simulink model "VDB_Unreal_ClosedLoop"  (R2026b)
settings: Solver=ode4  StopTime=35  FixedStep=0.02
undefined symbols (not defined in the file or in its folder): sih
libraries: sim3dlib x1, sim3dautolib x1, sim3dcameralib x1, autolibshared x1
settings Model: Creator=Hp  LastModifiedBy=Hp

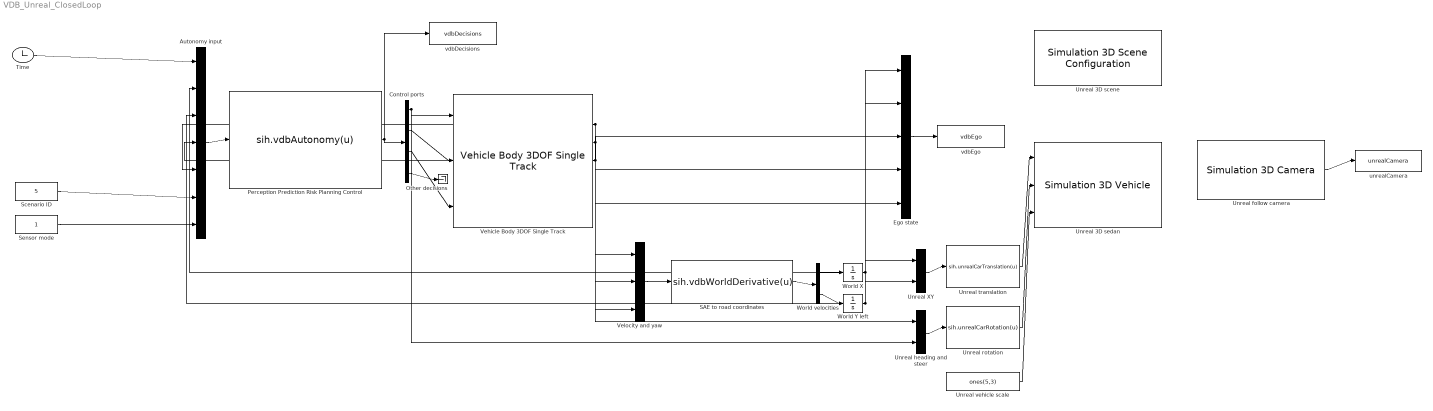
== system VDB_Unreal_ClosedLoop ==
  Autonomy input : Mux  Inputs=7
  Control ports : Demux  Outputs=[1 1 1 27]
  Ego state : Mux  Inputs=5
  Other decisions : Terminator
  Perception Prediction Risk Planning Control : MATLABFcn  MATLABFcn=sih.vdbAutonomy(u)  OutputDimensions=30  SampleTime=0.1
  SAE to road coordinates : MATLABFcn  MATLABFcn=sih.vdbWorldDerivative(u)  OutputDimensions=2  SampleTime=0.02
  Scenario ID : Constant  Value=5
  Sensor mode : Constant
  Time : Clock
  Unreal 3D scene : sim3dlib/Simulation 3D Scene Configuration  Priority=0  EnableWindow=on  ViewerType=Default Viewer  ProjectFormat=Default Scenes  SceneDesc=Open surface  ProjectName=C:\Program Files\MATLAB\R2026b\toolbox\shared\sim3d_projects\automotive_project_windows\UE\WindowsNoEditor\VehicleSimulation.exe  ScenePath=/Game/Maps/HwStrght  EnableOpenDRIVE=off  vehTagList={'Custom';'Scene Origin'}  vehTag=Custom  AttachedCameraRelativeTranslation=[0 0 0]  FreeCameraDefaultInitialTranslation=[-6, 0, 2]  AttachedCameraRelativeRotation=[0, -15, 0]  FreeCameraDefaultInitialRotation=[0, -15, 0]  ViewpointName=Custom  FreeCameraInitialTranslation=[0 0 0]  FreeCameraInitialRotation=[0 0 0]  OpVisEn=off  Ts=.02  EnableRemoteAccess=off  SimulationMode=CoSimulation  SimulateUsing=Interpreted execution  EnableAnimationRecording=off  OverrideDefaultRecording=off  AnimationRecordingFileName=sim3dAnimation.mat  AnimationRecordingInterval=[0 inf]  EnableWeather=off  SunAzimuth=90  SunAltitude=40.0  EnableGeospatialSun=off  Latitude=0  Longitude=0  Date=2023-01-01  Time=10:30:00  GeoTimeZone=-5.0  SunDaylightSaving=off  wind=1  clouds=10  EnableVolumetricClouds=off  CloudCoverage=0  CloudAltitude=6  fog=0  rain=0  RaindropsEffect=off  SnowDensity=0  EnableGeospatial=off  TilesetSource=Earth terrain  UseTrueOrigin=off  OriginHeight=200  OriginLatitude=40.744652  OriginLongitude=-73.988864  MapStyle=Aerial  AdditionalAssetIDs=[]  UseAdvancedSunSky=off  SolarTime=11  TimeZone=-5  Day=21  Month=9  Year=2022  UseDaylightSavingTime=on  DSTStartDay=10  DSTStartMonth=3  DSTEndDay=3  DSTEndMonth=11  DSTSwitchHour=2  sensorTag=MainCamera1  sensorId=1  sensorName=MainCamera1  mountLoc=Origin  offsetFlag=off  tmountOffset=[0, 0, 0]  rmountOffset=[0, 0, 0]  HorizontalResolution=1280  VerticalResolution=720  HorizontalFOV=60  mountPoint=[0 0 0]  mountOrientation=[0 0 0]  aMode=2  ID=1  GeoTrigger=Inactive  ViewNameList={'Custom'}  ViewTranslationList={'[0 0 0]'}  ViewRotationList={'[0 0 0]'}
      settings: LibrarySourceBlock=vehdynlibsim3dcore/Simulation 3D Scene Configuration
  Unreal 3D sedan : sim3dautolib/Simulation 3D Vehicle  Priority=-1  PassVehMesh=Sedan  MeshPath=/MathWorksAutomotiveContent/Vehicles/Muscle/Meshes/SK_MuscleCar.SK_MuscleCar  VehColor=Blue  ActorName=SIH_Ego  VehLightsControl=off  HeadlightColor=[ 1, 1, 1 ]  HighBeamIntensity=100000  LowBeamIntensity=60000  HighBeamConeAngle=1.22  LowBeamConeAngle=1.22  LeftHeadlightOrientation=[ 0, 0 ]  RightHeadlightOrientation=[ 0, 0 ]  BrakelightIntensity=500  ReverselightIntensity=500  SignallightIntensity=500  SignallightPeriod=1  SignalPulseWidth=50  Translation=zeros( 5, 3 )  Rotation=zeros( 5, 3 )  Scale=ones( 5, 3 )  SampleTime=0.02  ActorType=SimulinkVehicle  ID=C  aMode=2  ActorTag=SIH_Ego
      settings: LibrarySourceBlock=vehdynlibsim3d/Simulation 3D Vehicle
  Unreal XY : Mux  Inputs=2
  Unreal follow camera : sim3dcameralib/Simulation 3D Camera  Priority=1  sensorTag=Sim3dSensor  sensorId=1  sensorName=SIH_FollowCamera  vehTagList={'Custom ...';'SIH_Ego';'Scene Origin'}  vehTag=SIH_Ego  CoordinateSystem=ISO8855  mountLoc=Origin  offsetFlag=on  tmountOffset=[-8, 0, 3]  extTmount=off  rmountOffset=[0, 18, 0]  extRmount=off  FocalLength=[550, 550]  OpticalCenter=[320, 180]  ImageSize=[360, 640]  RadialDistortion=[0, 0]  TangentialDistortion=[0, 0]  SensorSkew=0  VisualizeFieldOfView=off  FieldOfViewRange=61  DepthOutportEnabled=off  SemanticOutportEnabled=off  TransformOutportEnabled=off  SampleTime=0.2  mountPoint=[-8 0 3]  mountOrientation=[0 18 0]  aMode=3  ID=1
      settings: LibrarySourceBlock=drivingsim3d/Simulation 3D Camera
  Unreal heading and steer : Mux  Inputs=2
  Unreal rotation : MATLABFcn  MATLABFcn=sih.unrealCarRotation(u)  OutputDimensions=[5 3]  Output1D=off  SampleTime=0.02
  Unreal translation : MATLABFcn  MATLABFcn=sih.unrealCarTranslation(u)  OutputDimensions=[5 3]  Output1D=off  SampleTime=0.02
  Unreal vehicle scale : Constant  Value=ones(5,3)
  Vehicle Body 3DOF Single Track : autolibshared/Vehicle Body 3DOF Single Track  trackMode=Single (bicycle)  inputMode=External longitudinal forces  frontSteerMode=on  rearSteerMode=off  extFMode=off  htchFMode=off  extMMode=off  htchMMode=off  windMode=off  extTamb=off  muMode=off  extGndPlnElev=off  extGndPlnRoll=off  extGndPlnPitch=off  extGndPlnDCM=off  extXo=off  extxdoto=off  extYo=off  extydoto=off  extpsio=off  extro=off  aMode=2  NF=2  NR=2  m=2000  a=1.35  b=1.35  h=0.35  dh=1  hh=0.2  X_o=0  xdot_o=0  d=0  hl=0  w=[1.4,1.4]  CalphaMode=Constant  sigmaMode=on  sigma_f=.1  sigma_r=.1  Cy_f=12e3  Cy_r=11e3  Cy_f_data="[1.396121365092108e+04\t4.232462640127975e+04\t6.754894575573687e+04\t8.835784428391886e+04\t1.043551700699839e+05\t1.158335754468729e+05\t1.234691551560788e+05\t1.280575366661118e+05\t1.298126639907242e+05\t1.298126639907242e+05]"  alpha_f_brk=[-0.785, -0.628, -0.471, -0.314, -0.157, 0.000, 0.157, 0.314, 0.471, 0.628, 0.785]  Fz_f_brk="[500\t1.555555555555556e+03\t2.611111111111111e+03\t3.666666666666667e+03\t4.722222222222223e+03\t5.777777777777777e+03\t6.833333333333333e+03\t7.888888888888889e+03\t8.944444444444445e+03\t10000]"  Cy_r_data="[1.396121365092108e+04\t4.232462640127975e+04\t6.754894575573687e+04\t8.835784428391886e+04\t1.043551700699839e+05\t1.158335754468729e+05\t1.234691551560788e+05\t1.280575366661118e+05\t1.298126639907242e+05\t1.298126639907242e+05]"  alpha_r_brk=[-0.785, -0.628, -0.471, -0.314, -0.157, 0.000, 0.157, 0.314, 0.471, 0.628, 0.785]  Fz_r_brk="[500\t1.555555555555556e+03\t2.611111111111111e+03\t3.666666666666667e+03\t4.722222222222223e+03\t5.777777777777777e+03\t6.833333333333333e+03\t7.888888888888889e+03\t8.944444444444445e+03\t10000]"  Fznom=5000  Y_o=0  ydot_o=0  Izz=4000  psi_o=0  r_o=0  Af=2  Cd=.3  Cl=.1  Cpm=.1  beta_w=[0,0.1745,0.3491,0.5236,0.6981,0.8727,1.0472,1.2217,1.3963,1.5708]  Cs=[0.1000,0.1000,0.1000,0.1000,0.1000,0.1000,0.1000,0.1000,0.1000,0.1000]  Cym=[0,0,0.0667,0.1000,0.1333,0.1667,0.2000,0.2333,0.2667,0.3000]  Pabs=101325  Tair=273  g=9.81  mu=1  GndPlnRoll=0  GndPlnPitch=0  GndPlnElev=0  xdot_tol=0.1  Fxtire_sat=7e4  Fytire_sat=7e4  longOff=0  latOff=0  vertOff=0.35  wrapAng=off
  Velocity and yaw : Mux  Inputs=3
  World X : Integrator
  World Y left : Integrator
  World velocities : Demux  Outputs=2
  unrealCamera : ToWorkspace  VariableName=unrealCamera  SaveFormat=Timeseries  SampleTime=-1
  vdbDecisions : ToWorkspace  VariableName=vdbDecisions  SaveFormat=Timeseries  SampleTime=-1
  vdbEgo : ToWorkspace  VariableName=vdbEgo  SaveFormat=Timeseries  SampleTime=-1
  wires:
  Time/1 -> Autonomy input/1
  World X/1 -> Autonomy input/2, Ego state/1, Unreal XY/1
  World Y left/1 -> Autonomy input/3, Ego state/2, Unreal XY/2
  Vehicle Body 3DOF Single Track/4 -> Autonomy input/4, Velocity and yaw/3, Ego state/3, Unreal heading and steer/1
  Vehicle Body 3DOF Single Track/2 -> Autonomy input/5, Velocity and yaw/1, Ego state/4
  Scenario ID/1 -> Autonomy input/6
  Sensor mode/1 -> Autonomy input/7
  Autonomy input/1 -> Perception Prediction Risk Planning Control/1
  Perception Prediction Risk Planning Control/1 -> Control ports/1, vdbDecisions/1
  Control ports/1 -> Vehicle Body 3DOF Single Track/1, Unreal heading and steer/2
  Control ports/2 -> Vehicle Body 3DOF Single Track/2
  Control ports/3 -> Vehicle Body 3DOF Single Track/3
  Control ports/4 -> Other decisions/1
  Vehicle Body 3DOF Single Track/3 -> Velocity and yaw/2, Ego state/5
  Velocity and yaw/1 -> SAE to road coordinates/1
  SAE to road coordinates/1 -> World velocities/1
  World velocities/1 -> World X/1
  World velocities/2 -> World Y left/1
  Ego state/1 -> vdbEgo/1
  Unreal XY/1 -> Unreal translation/1
  Unreal translation/1 -> Unreal 3D sedan/1
  Unreal heading and steer/1 -> Unreal rotation/1
  Unreal rotation/1 -> Unreal 3D sedan/2
  Unreal vehicle scale/1 -> Unreal 3D sedan/3
  Unreal follow camera/1 -> unrealCamera/1
